simulink model "SinglePhFullControlledConverter"  (R2013a)
settings: Solver=ode45  StartTime=0.0  StopTime=4  RelTol=1e-3
libraries: powerlib x14
settings Model: Creator=avirup  LastModifiedBy=avirup

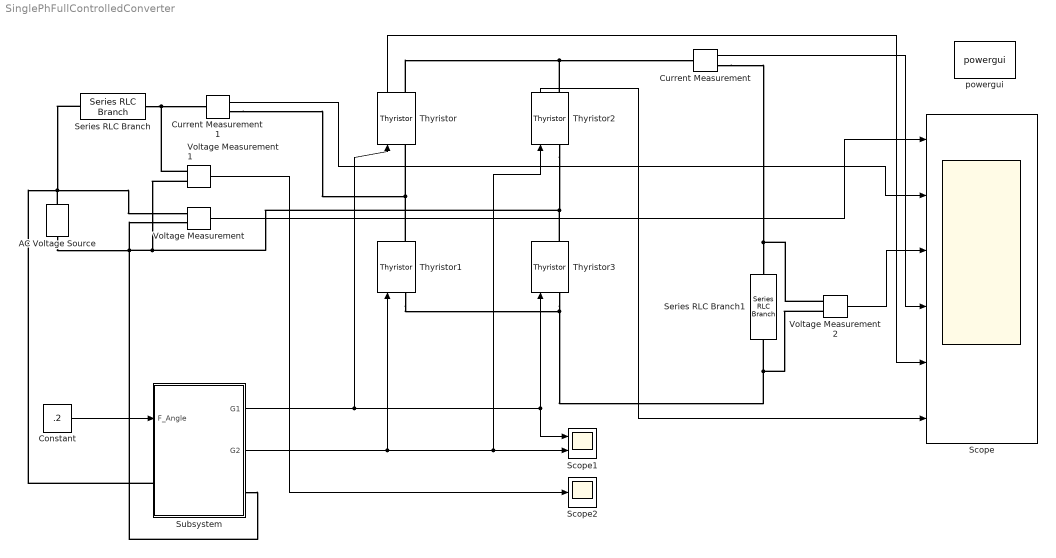
== system SinglePhFullControlledConverter ==
  AC Voltage Source : powerlib/Electrical Sources/AC Voltage Source  Amplitude=100  Phase=0  Frequency=50  SampleTime=0  Measurements=None
  Constant : Constant  Value=.2
  Current Measurement : powerlib/Measurements/Current Measurement  PhasorSimulation=off  OutputType=Complex  PSBequivalent=0
  Current Measurement1 : powerlib/Measurements/Current Measurement  PhasorSimulation=off  OutputType=Complex  PSBequivalent=0
  Scope : Scope  NumInputPorts=6
      settings: YMin=-100~-100~-50~-10~-125~-125  YMax=100~100~125~100~100~100  SaveName=ScopeData3
  Scope1 : Scope  NumInputPorts=2
      settings: YMin=-5~-5  YMax=5~5  SaveName=ScopeData4
  Scope2 : Scope
      settings: SaveName=ScopeData5
  Series RLC Branch : powerlib/Elements/Series RLC Branch  LConnTagsString=__new0  RConnTagsString=__new0  BranchType=L  Resistance=1  Inductance=.5e-3  SetiL0=off  InitialCurrent=0  Capacitance=1e-6  Setx0=off  InitialVoltage=0  Measurements=None
  Series RLC Branch1 : powerlib/Elements/Series RLC Branch  LConnTagsString=__new0  RConnTagsString=__new0  BranchType=RL  Resistance=1  Inductance=.5e-3  SetiL0=off  InitialCurrent=0  Capacitance=1e-6  Setx0=off  InitialVoltage=0  Measurements=None
  Subsystem : Subsystem
  Thyristor{,1..3} (4 alike) : powerlib/Power Electronics/Thyristor  Ron=0.001  Lon=0  Vf=0.8  IC=0  Rs=500  Cs=250e-9  Measurements=on
  Voltage Measurement : powerlib/Measurements/Voltage Measurement  PhasorSimulation=off  OutputType=Complex  PSBequivalent=0
  Voltage Measurement1 : powerlib/Measurements/Voltage Measurement  PhasorSimulation=off  OutputType=Complex  PSBequivalent=0
  Voltage Measurement2 : powerlib/Measurements/Voltage Measurement  PhasorSimulation=off  OutputType=Complex  PSBequivalent=0
  powergui : powerlib/powergui  Priority=1  SimulationMode=Continuous  SolverType=Tustin  SampleTime=50e-6  frequency=60  SPID=off  DisableSnubberDevices=off  DisableRonSwitches=off  DisableVfSwitches=off  SwTol=0  Interpol=off  DisplayEquations=off  frequencyindice=50  Pbase=100e6  ErrMax=1e-4  Iterations=50  UnitsV=kV  UnitsW=MW  FunctionMessages=off  echomessages=off  HookPort=off  EnableUseOfTLC=off  x0status=blocks  RestoreLinks=warning  ResistiveCurrentMeasurement=off  Frange=[0:2:500]  Ylog=off  Xlog=on  ShowGrid=off  save=off  variable=ZData  ZoomFFT=off  StartTime=0.0  cycles=1  DisplayStyle=1  fundamental=60  FreqAxis=off  MaxFrequency=1000  frequencyindicesteady=1  RmsSteady=1  display=off  Ts=0  methode=off
  wires:
  Constant/1 -> Subsystem/1(F_Angle)
  Subsystem/1(G1) -> Scope1/1, Thyristor3/1, Thyristor/1
  Subsystem/2(G2) -> Thyristor1/1, Thyristor2/1, Scope1/2
  Voltage Measurement1/1 -> Scope2/1
  Voltage Measurement/1 -> Scope/1
  Current Measurement1/1 -> Scope/2
  Voltage Measurement2/1 -> Scope/3
  Current Measurement/1 -> Scope/4
  Thyristor/1 -> Scope/5
  Thyristor2/1 -> Scope/6
  connections:
  AC Voltage Source/RConn1 -- Series RLC Branch/LConn1 -- Subsystem/LConn1 -- Voltage Measurement/LConn1
  AC Voltage Source/LConn1 -- Thyristor2/LConn1 -- Thyristor3/RConn1 -- Voltage Measurement1/LConn2 -- Subsystem/RConn1 -- Voltage Measurement/LConn2
  Thyristor1/RConn1 -- Current Measurement1/RConn1 -- Thyristor/LConn1
  Series RLC Branch/RConn1 -- Current Measurement1/LConn1 -- Voltage Measurement1/LConn1
  Thyristor2/RConn1 -- Current Measurement/LConn1 -- Thyristor/RConn1
  Current Measurement/RConn1 -- Voltage Measurement2/LConn1 -- Series RLC Branch1/LConn1
  Thyristor3/LConn1 -- Thyristor1/LConn1 -- Voltage Measurement2/LConn2 -- Series RLC Branch1/RConn1

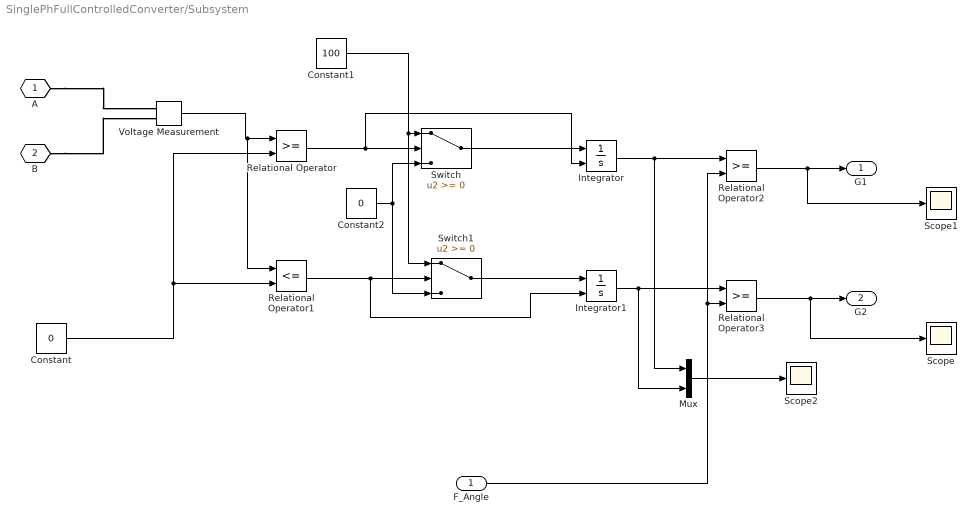
== system SinglePhFullControlledConverter/Subsystem ==
  F_Angle : Inport
  Constant : Constant  Value=0
  Constant1 : Constant  Value=100
  Constant2 : Constant  Value=0
  Integrator : Integrator  ExternalReset=falling
  Integrator1 : Integrator  ExternalReset=falling
  Mux : Mux  Inputs=2
  Relational Operator : RelationalOperator  OutDataTypeStr=boolean
  Relational Operator1 : RelationalOperator  Operator=<=  OutDataTypeStr=boolean
  Relational Operator2 : RelationalOperator  OutDataTypeStr=boolean
  Relational Operator3 : RelationalOperator  OutDataTypeStr=boolean
  Scope : Scope
  Scope1 : Scope
  Scope2 : Scope
      settings: SaveName=ScopeData2
  Switch : Switch
  Switch1 : Switch
  Voltage Measurement : powerlib/Measurements/Voltage Measurement  PhasorSimulation=off  OutputType=Complex  PSBequivalent=0
  A : PMIOPort  Tag=PMCPort  Port=1  Side=Left
  B : PMIOPort  Tag=PMCPort  Port=2  Side=Right
  G1 : Outport
  G2 : Outport  Port=2
  wires:
  Relational Operator1/1 -> Switch1/2, Integrator1/2
  Switch/1 -> Integrator/1
  Relational Operator3/1 -> G2/1, Scope/1
  Constant/1 -> Relational Operator1/2, Relational Operator/2
  Voltage Measurement/1 -> Relational Operator1/1, Relational Operator/1
  Relational Operator2/1 -> G1/1, Scope1/1
  Constant2/1 -> Switch1/3, Switch/3
  Relational Operator/1 -> Switch/2, Integrator/2
  F_Angle/1 -> Relational Operator3/2, Relational Operator2/2
  Switch1/1 -> Integrator1/1
  Integrator/1 -> Relational Operator2/1, Mux/1
  Constant1/1 -> Switch1/1, Switch/1
  Integrator1/1 -> Relational Operator3/1, Mux/2
  Mux/1 -> Scope2/1
  connections:
  B/RConn1 -- Voltage Measurement/LConn2
  A/RConn1 -- Voltage Measurement/LConn1
